simulink model "calculator"  (R2014a)
settings: Solver=VariableStepAuto  StartTime=0.0  StopTime=10.0  RelTol=1e-3
libraries: hdlsllib x43
(part 1 of 4)
settings Model: Creator=Ray  LastModifiedBy=you.r
settings DataIOCC: LimitDataPoints=off  SaveFormat=Dataset
settings OptimizationCC: LifeSpan=auto  SimCompilerOptimization=off
settings DebuggingCC: MergeDetectMultiDrivingBlocksExec=error  SolverPrmCheckMsg=none  FcnCallInpInsideContextMsg=error  FrameProcessingCompatibilityMsg=error  SFUnexpectedBacktrackingDiag=error  SFNoUnconditionalDefaultTransitionDiag=error
settings HardwareCC: ProdBitPerPointer=64  ProdLargestAtomicFloat=Float  ProdIntDivRoundTo=Zero  ProdEndianess=LittleEndian  ProdWordSize=64  ProdHWDeviceType=Intel->x86-64 (Windows64)
settings ModelReferenceCC: PropagateSignalLabelsOutOfModel=on
settings RTWCC: RTWCompilerOptimization=off
settings GRTTargetCC: TargetLangStandard=C99 (ISO)  GeneratePreprocessorConditionals=Use local settings

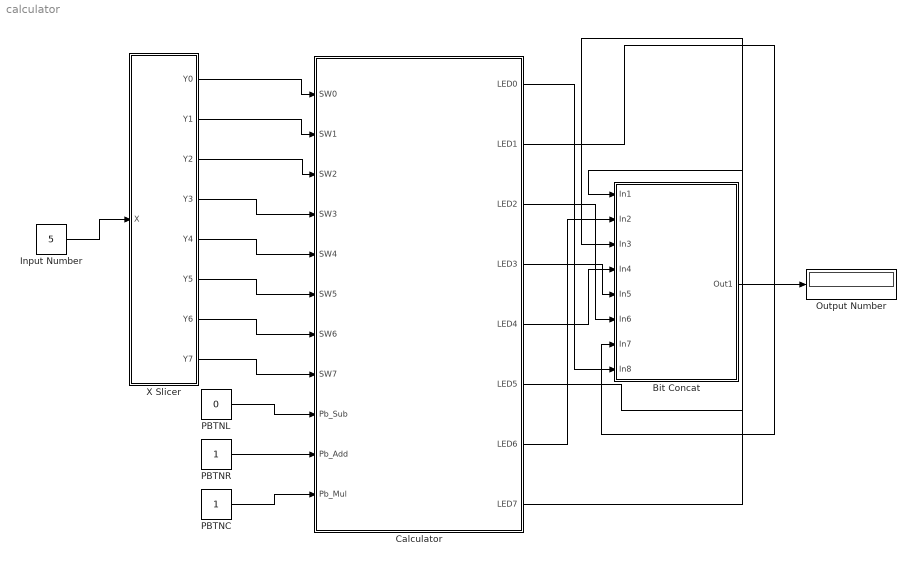
== system calculator ==
  Bit Concat : Subsystem
  Calculator : Subsystem  TreatAsAtomicUnit=on
  Input Number : Constant  Value=5  OutDataTypeStr=uint8  SampleTime=-1
  Output Number : Display
  PBTNC : Constant  OutDataTypeStr=boolean  SampleTime=1
  PBTNL : Constant  Value=0  OutDataTypeStr=boolean  SampleTime=1
  PBTNR : Constant  OutDataTypeStr=boolean  SampleTime=1
  X Slicer : Subsystem
  wires:
  Input Number/1 -> X Slicer/1(X)
  X Slicer/8(Y7) -> Calculator/8(SW7)
  X Slicer/7(Y6) -> Calculator/7(SW6)
  X Slicer/6(Y5) -> Calculator/6(SW5)
  X Slicer/5(Y4) -> Calculator/5(SW4)
  X Slicer/4(Y3) -> Calculator/4(SW3)
  X Slicer/3(Y2) -> Calculator/3(SW2)
  X Slicer/2(Y1) -> Calculator/2(SW1)
  X Slicer/1(Y0) -> Calculator/1(SW0)
  Calculator/8(LED7) -> Bit Concat/1(In1)
  Calculator/1(LED0) -> Bit Concat/8(In8)
  Calculator/2(LED1) -> Bit Concat/7(In7)
  Calculator/3(LED2) -> Bit Concat/6(In6)
  Calculator/4(LED3) -> Bit Concat/5(In5)
  Calculator/5(LED4) -> Bit Concat/4(In4)
  Calculator/6(LED5) -> Bit Concat/3(In3)
  Calculator/7(LED6) -> Bit Concat/2(In2)
  Bit Concat/1(Out1) -> Output Number/1
  PBTNR/1 -> Calculator/10(Pb_Add)
  PBTNC/1 -> Calculator/11(Pb_Mul)
  PBTNL/1 -> Calculator/9(Pb_Sub)

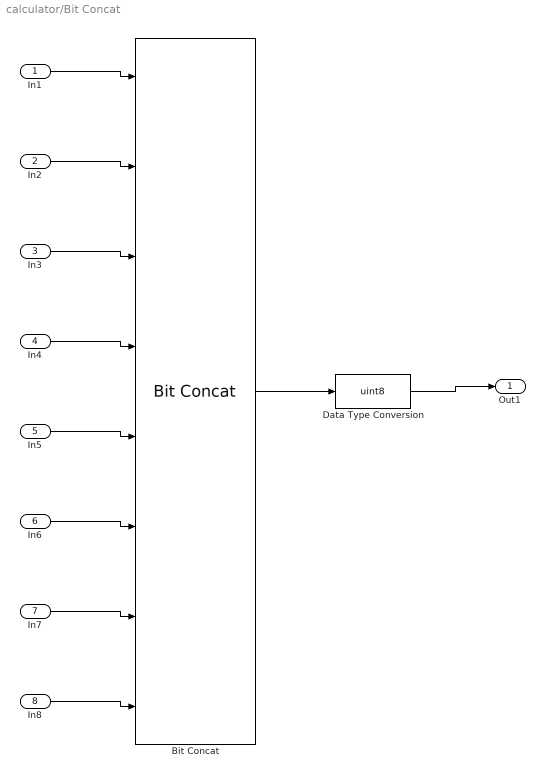
== system calculator/Bit Concat ==
  In1 : Inport
  In2 : Inport  Port=2
  In3 : Inport  Port=3
  In4 : Inport  Port=4
  In5 : Inport  Port=5
  In6 : Inport  Port=6
  In7 : Inport  Port=7
  In8 : Inport  Port=8
  Bit Concat : hdlsllib/HDL Operations/Bit Concat  numInputs=8
  Data Type Conversion : DataTypeConversion  OutDataTypeStr=uint8
  Out1 : Outport  OutDataTypeStr=uint8
  wires:
  Data Type Conversion/1 -> Out1/1
  Bit Concat/1 -> Data Type Conversion/1
  In6/1 -> Bit Concat/6
  In8/1 -> Bit Concat/8
  In1/1 -> Bit Concat/1
  In3/1 -> Bit Concat/3
  In5/1 -> Bit Concat/5
  In7/1 -> Bit Concat/7
  In4/1 -> Bit Concat/4
  In2/1 -> Bit Concat/2

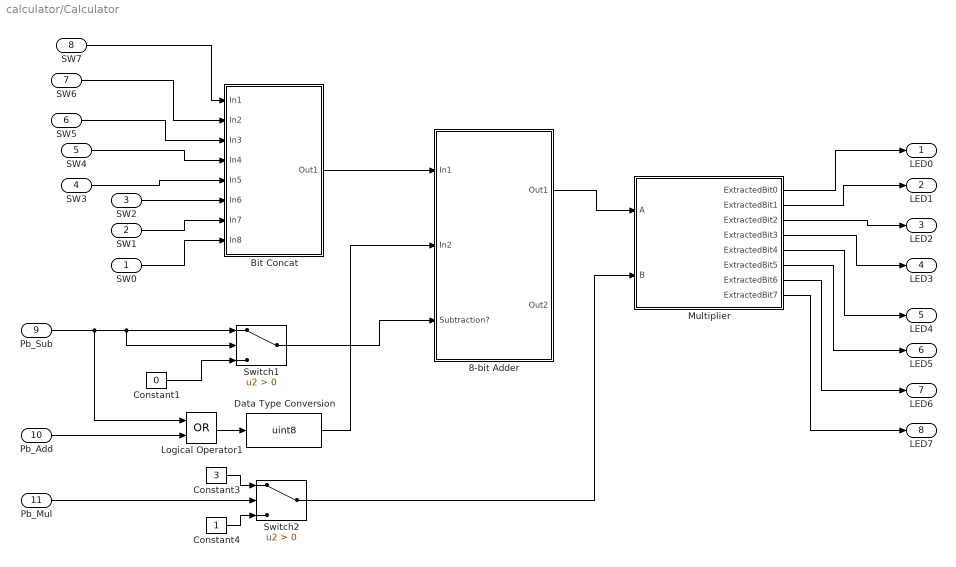
== system calculator/Calculator ==
  SW0 : Inport  OutDataTypeStr=boolean  SampleTime=1
  SW1 : Inport  Port=2  OutDataTypeStr=boolean  SampleTime=1
  SW2 : Inport  Port=3  OutDataTypeStr=boolean  SampleTime=1
  SW3 : Inport  Port=4  OutDataTypeStr=boolean  SampleTime=1
  SW4 : Inport  Port=5  OutDataTypeStr=boolean  SampleTime=1
  SW5 : Inport  Port=6  OutDataTypeStr=boolean  SampleTime=1
  SW6 : Inport  Port=7  OutDataTypeStr=boolean  SampleTime=1
  SW7 : Inport  Port=8  OutDataTypeStr=boolean  SampleTime=1
  Pb_Sub : Inport  Port=9  OutDataTypeStr=boolean  SampleTime=1
  Pb_Add : Inport  Port=10  OutDataTypeStr=boolean  SampleTime=1
  Pb_Mul : Inport  Port=11  OutDataTypeStr=boolean  SampleTime=1
  8-bit Adder : Subsystem
  Bit Concat : Subsystem
  Constant1 : Constant  Value=0  OutDataTypeStr=boolean  SampleTime=1
  Constant3 : Constant  Value=3  OutDataTypeStr=uint8  SampleTime=1
  Constant4 : Constant  OutDataTypeStr=boolean  SampleTime=1
  Data Type Conversion : DataTypeConversion  OutDataTypeStr=uint8
  Logical Operator1 : Logic  Operator=OR  AllPortsSameDT=off  OutDataTypeStr=boolean
  Multiplier : Subsystem
  Switch1 : Switch  Criteria=u2 > Threshold
  Switch2 : Switch  Criteria=u2 > Threshold  OutDataTypeStr=uint8
  LED0 : Outport  SampleTime=1
  LED1 : Outport  Port=2  SampleTime=1
  LED2 : Outport  Port=3  SampleTime=1
  LED3 : Outport  Port=4  SampleTime=1
  LED4 : Outport  Port=5  SampleTime=1
  LED5 : Outport  Port=6  SampleTime=1
  LED6 : Outport  Port=7  SampleTime=1
  LED7 : Outport  Port=8  SampleTime=1
  wires:
  Pb_Sub/1 -> Switch1/2, Switch1/1, Logical Operator1/1
  Pb_Mul/1 -> Switch2/2
  Pb_Add/1 -> Logical Operator1/2
  Bit Concat/1(Out1) -> 8-bit Adder/1(In1)
  Constant3/1 -> Switch2/1
  Switch2/1 -> Multiplier/2(B)
  Constant4/1 -> Switch2/3
  Constant1/1 -> Switch1/3
  Data Type Conversion/1 -> 8-bit Adder/2(In2)
  Logical Operator1/1 -> Data Type Conversion/1
  Multiplier/2(ExtractedBit1) -> LED1/1
  Multiplier/3(ExtractedBit2) -> LED2/1
  Multiplier/1(ExtractedBit0) -> LED0/1
  Multiplier/4(ExtractedBit3) -> LED3/1
  Multiplier/5(ExtractedBit4) -> LED4/1
  Multiplier/7(ExtractedBit6) -> LED6/1
  Multiplier/6(ExtractedBit5) -> LED5/1
  Multiplier/8(ExtractedBit7) -> LED7/1
  Switch1/1 -> 8-bit Adder/3("Subtraction? ")
  8-bit Adder/1(Out1) -> Multiplier/1(A)
  SW2/1 -> Bit Concat/6(In6)
  SW3/1 -> Bit Concat/5(In5)
  SW1/1 -> Bit Concat/7(In7)
  SW0/1 -> Bit Concat/8(In8)
  SW4/1 -> Bit Concat/4(In4)
  SW5/1 -> Bit Concat/3(In3)
  SW6/1 -> Bit Concat/2(In2)
  SW7/1 -> Bit Concat/1(In1)

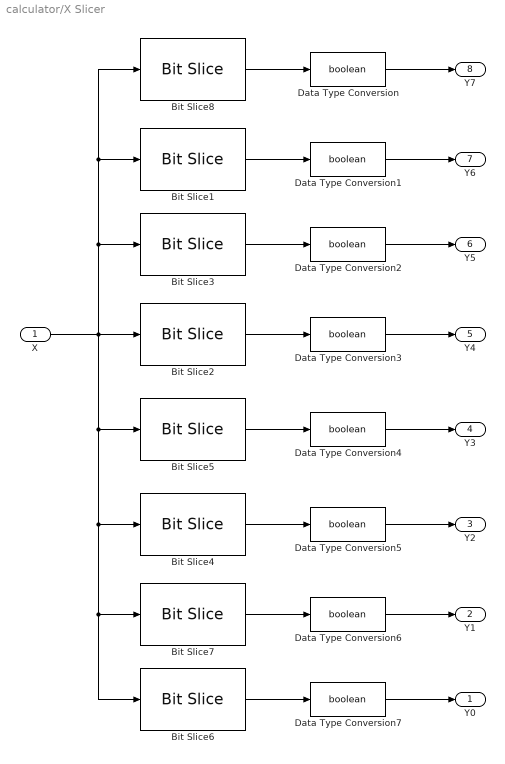
== system calculator/X Slicer ==
  X : Inport  OutDataTypeStr=uint8  SampleTime=1
  Bit Slice1 : hdlsllib/HDL Operations/Bit Slice  lidx=6  ridx=6
  Bit Slice2 : hdlsllib/HDL Operations/Bit Slice  lidx=4  ridx=4
  Bit Slice3 : hdlsllib/HDL Operations/Bit Slice  lidx=5  ridx=5
  Bit Slice4 : hdlsllib/HDL Operations/Bit Slice  lidx=2  ridx=2
  Bit Slice5 : hdlsllib/HDL Operations/Bit Slice  lidx=3  ridx=3
  Bit Slice6 : hdlsllib/HDL Operations/Bit Slice  lidx=0  ridx=0
  Bit Slice7 : hdlsllib/HDL Operations/Bit Slice  lidx=1  ridx=1
  Bit Slice8 : hdlsllib/HDL Operations/Bit Slice  lidx=7  ridx=7
  Data Type Conversion{,1..7} (8 alike) : DataTypeConversion  OutDataTypeStr=boolean
  Y0 : Outport
  Y1 : Outport  Port=2
  Y2 : Outport  Port=3
  Y3 : Outport  Port=4
  Y4 : Outport  Port=5
  Y5 : Outport  Port=6
  Y6 : Outport  Port=7
  Y7 : Outport  Port=8
  wires:
  X/1 -> Bit Slice2/1, Bit Slice5/1, Bit Slice4/1, Bit Slice7/1, Bit Slice6/1, Bit Slice3/1, Bit Slice1/1, Bit Slice8/1
  Data Type Conversion/1 -> Y7/1
  Data Type Conversion1/1 -> Y6/1
  Bit Slice3/1 -> Data Type Conversion2/1
  Bit Slice2/1 -> Data Type Conversion3/1
  Bit Slice5/1 -> Data Type Conversion4/1
  Data Type Conversion6/1 -> Y1/1
  Bit Slice8/1 -> Data Type Conversion/1
  Bit Slice1/1 -> Data Type Conversion1/1
  Bit Slice7/1 -> Data Type Conversion6/1
  Data Type Conversion7/1 -> Y0/1
  Bit Slice6/1 -> Data Type Conversion7/1
  Bit Slice4/1 -> Data Type Conversion5/1
  Data Type Conversion2/1 -> Y5/1
  Data Type Conversion3/1 -> Y4/1
  Data Type Conversion4/1 -> Y3/1
  Data Type Conversion5/1 -> Y2/1

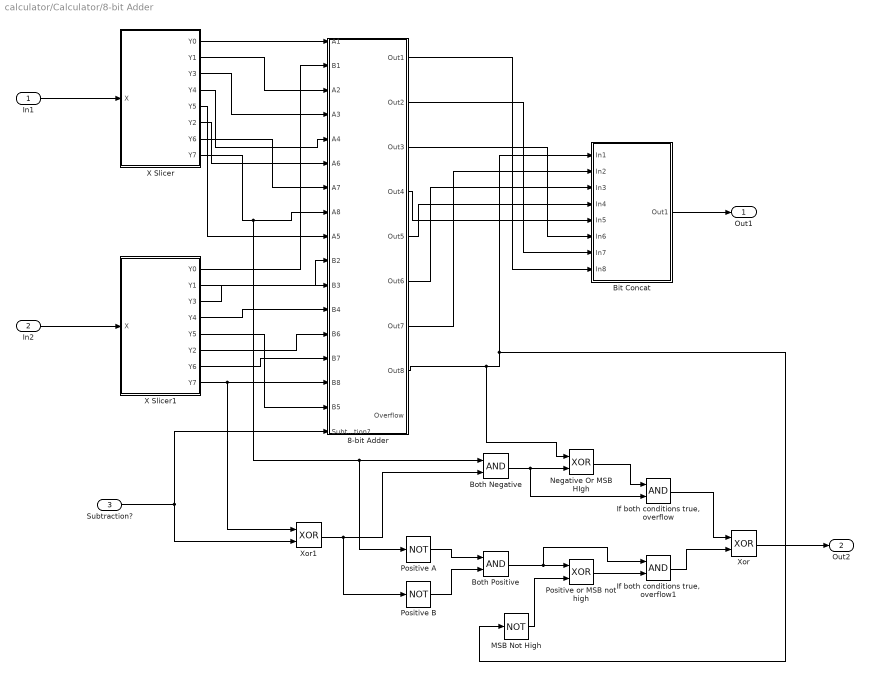
== system calculator/Calculator/8-bit Adder ==
  In1 : Inport  OutDataTypeStr=uint8
  In2 : Inport  Port=2  OutDataTypeStr=uint8
  "Subtraction? " : Inport  Port=3
  8-bit Adder : Subsystem
  Bit Concat : Subsystem
  Both Negative : Logic  AllPortsSameDT=off  OutDataTypeStr=boolean
  Both Positive : Logic  AllPortsSameDT=off  OutDataTypeStr=boolean
  "If both conditions true, overflow" : Logic  AllPortsSameDT=off  OutDataTypeStr=boolean
  "If both conditions true, overflow1" : Logic  AllPortsSameDT=off  OutDataTypeStr=boolean
  MSB Not High : Logic  Operator=NOT  AllPortsSameDT=off  OutDataTypeStr=boolean
  Negative Or MSB HIgh : Logic  Operator=XOR  AllPortsSameDT=off  OutDataTypeStr=boolean
  Positive A : Logic  Operator=NOT  AllPortsSameDT=off  OutDataTypeStr=boolean
  Positive B : Logic  Operator=NOT  AllPortsSameDT=off  OutDataTypeStr=boolean
  Positive or MSB not high : Logic  Operator=XOR  AllPortsSameDT=off  OutDataTypeStr=boolean
  X Slicer : Subsystem
  X Slicer1 : Subsystem
  Xor : Logic  Operator=XOR  AllPortsSameDT=off  OutDataTypeStr=boolean
  Xor1 : Logic  Operator=XOR  AllPortsSameDT=off  OutDataTypeStr=boolean
  Out1 : Outport
  Out2 : Outport  Port=2
  wires:
  Bit Concat/1(Out1) -> Out1/1
  In1/1 -> X Slicer/1(X)
  In2/1 -> X Slicer1/1(X)
  8-bit Adder/8(Out8) -> Negative Or MSB HIgh/1, MSB Not High/1, Bit Concat/1(In1)
  8-bit Adder/7(Out7) -> Bit Concat/2(In2)
  8-bit Adder/6(Out6) -> Bit Concat/3(In3)
  8-bit Adder/5(Out5) -> Bit Concat/4(In4)
  8-bit Adder/4(Out4) -> Bit Concat/5(In5)
  8-bit Adder/3(Out3) -> Bit Concat/6(In6)
  8-bit Adder/2(Out2) -> Bit Concat/7(In7)
  8-bit Adder/1(Out1) -> Bit Concat/8(In8)
  X Slicer/1(Y0) -> 8-bit Adder/1(A1)
  X Slicer/2(Y1) -> 8-bit Adder/3(A2)
  X Slicer/3(Y3) -> 8-bit Adder/4(A3)
  X Slicer/4(Y4) -> 8-bit Adder/5(A4)
  X Slicer/5(Y5) -> 8-bit Adder/9(A5)
  X Slicer/6(Y2) -> 8-bit Adder/6(A6)
  X Slicer/7(Y6) -> 8-bit Adder/7(A7)
  X Slicer1/1(Y0) -> 8-bit Adder/2(B1)
  X Slicer1/2(Y1) -> 8-bit Adder/10(B2)
  X Slicer1/3(Y3) -> 8-bit Adder/11(B3)
  X Slicer1/4(Y4) -> 8-bit Adder/12(B4)
  X Slicer1/5(Y5) -> 8-bit Adder/16(B5)
  X Slicer1/6(Y2) -> 8-bit Adder/13(B6)
  X Slicer1/7(Y6) -> 8-bit Adder/14(B7)
  X Slicer1/8(Y7) -> Xor1/1, 8-bit Adder/15(B8)
  Both Negative/1 -> "If both conditions true, overflow"/2, Negative Or MSB HIgh/2
  Negative Or MSB HIgh/1 -> "If both conditions true, overflow"/1
  X Slicer/8(Y7) -> Positive A/1, Both Negative/1, 8-bit Adder/8(A8)
  Positive A/1 -> Both Positive/1
  Positive B/1 -> Both Positive/2
  Both Positive/1 -> "If both conditions true, overflow1"/1, Positive or MSB not high/1
  MSB Not High/1 -> Positive or MSB not high/2
  Positive or MSB not high/1 -> "If both conditions true, overflow1"/2
  Xor/1 -> Out2/1
  "If both conditions true, overflow1"/1 -> Xor/2
  "If both conditions true, overflow"/1 -> Xor/1
  "Subtraction? "/1 -> 8-bit Adder/17(Subtraction?), Xor1/2
  Xor1/1 -> Positive B/1, Both Negative/2

== system calculator/Calculator/Bit Concat ==
  In1 : Inport
  In2 : Inport  Port=2
  In3 : Inport  Port=3
  In4 : Inport  Port=4
  In5 : Inport  Port=5
  In6 : Inport  Port=6
  In7 : Inport  Port=7
  In8 : Inport  Port=8
  Bit Concat1 : hdlsllib/HDL Operations/Bit Concat  numInputs=8
  Data Type Conversion : DataTypeConversion  OutDataTypeStr=uint8
  Out1 : Outport  OutDataTypeStr=uint8
  wires:
  Data Type Conversion/1 -> Out1/1
  Bit Concat1/1 -> Data Type Conversion/1
  In5/1 -> Bit Concat1/5
  In6/1 -> Bit Concat1/6
  In4/1 -> Bit Concat1/4
  In3/1 -> Bit Concat1/3
  In7/1 -> Bit Concat1/7
  In8/1 -> Bit Concat1/8
  In2/1 -> Bit Concat1/2
  In1/1 -> Bit Concat1/1

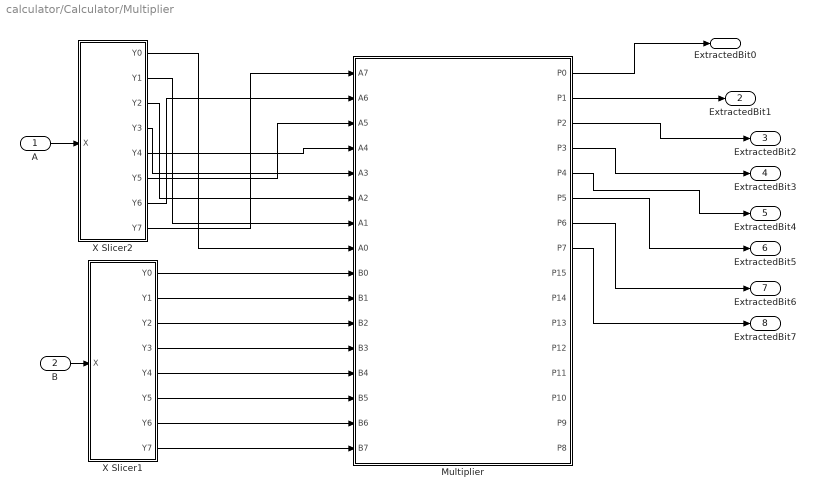
== system calculator/Calculator/Multiplier ==
  A : Inport  OutDataTypeStr=uint8
  B : Inport  Port=2  OutDataTypeStr=uint8
  Multiplier : Subsystem
  X Slicer1 : Subsystem
  X Slicer2 : Subsystem
  ExtractedBit0 : Outport  SampleTime=1
  ExtractedBit1 : Outport  Port=2  SampleTime=1
  ExtractedBit2 : Outport  Port=3  SampleTime=1
  ExtractedBit3 : Outport  Port=4  SampleTime=1
  ExtractedBit4 : Outport  Port=5  SampleTime=1
  ExtractedBit5 : Outport  Port=6  SampleTime=1
  ExtractedBit6 : Outport  Port=7  SampleTime=1
  ExtractedBit7 : Outport  Port=8  SampleTime=1
  wires:
  B/1 -> X Slicer1/1(X)
  A/1 -> X Slicer2/1(X)
  X Slicer1/1(Y0) -> Multiplier/9(B0)
  X Slicer1/2(Y1) -> Multiplier/10(B1)
  X Slicer1/3(Y2) -> Multiplier/11(B2)
  X Slicer1/4(Y3) -> Multiplier/12(B3)
  X Slicer1/5(Y4) -> Multiplier/13(B4)
  X Slicer1/6(Y5) -> Multiplier/14(B5)
  X Slicer1/7(Y6) -> Multiplier/15(B6)
  X Slicer1/8(Y7) -> Multiplier/16(B7)
  Multiplier/1(P0) -> ExtractedBit0/1
  Multiplier/2(P1) -> ExtractedBit1/1
  Multiplier/3(P2) -> ExtractedBit2/1
  Multiplier/4(P3) -> ExtractedBit3/1
  Multiplier/5(P4) -> ExtractedBit4/1
  Multiplier/6(P5) -> ExtractedBit5/1
  Multiplier/7(P6) -> ExtractedBit6/1
  Multiplier/8(P7) -> ExtractedBit7/1
  X Slicer2/8(Y7) -> Multiplier/1(A7)
  X Slicer2/1(Y0) -> Multiplier/8(A0)
  X Slicer2/2(Y1) -> Multiplier/7(A1)
  X Slicer2/3(Y2) -> Multiplier/6(A2)
  X Slicer2/4(Y3) -> Multiplier/5(A3)
  X Slicer2/5(Y4) -> Multiplier/4(A4)
  X Slicer2/6(Y5) -> Multiplier/3(A5)
  X Slicer2/7(Y6) -> Multiplier/2(A6)

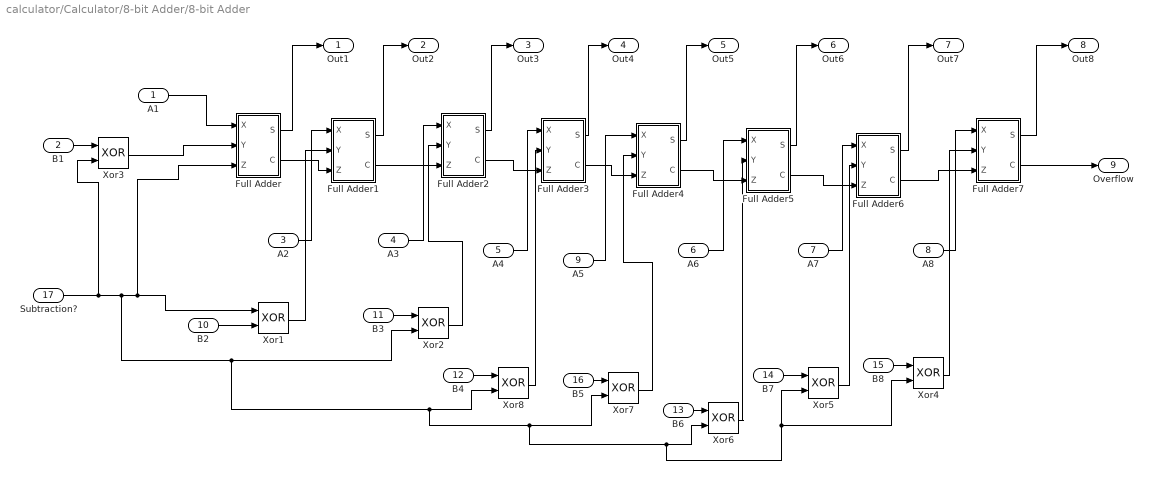
== system calculator/Calculator/8-bit Adder/8-bit Adder ==
  A1 : Inport
  B1 : Inport  Port=2
  A2 : Inport  Port=3
  A3 : Inport  Port=4
  A4 : Inport  Port=5
  A6 : Inport  Port=6
  A7 : Inport  Port=7
  A8 : Inport  Port=8
  A5 : Inport  Port=9
  B2 : Inport  Port=10
  B3 : Inport  Port=11
  B4 : Inport  Port=12
  B6 : Inport  Port=13
  B7 : Inport  Port=14
  B8 : Inport  Port=15
  B5 : Inport  Port=16
  Subtraction? : Inport  Port=17  OutDataTypeStr=boolean
  Full Adder : Subsystem
  Full Adder1 : Subsystem
  Full Adder2 : Subsystem
  Full Adder3 : Subsystem
  Full Adder4 : Subsystem
  Full Adder5 : Subsystem
  Full Adder6 : Subsystem
  Full Adder7 : Subsystem
  Xor{1..8} (8 alike) : Logic  Operator=XOR  AllPortsSameDT=off  OutDataTypeStr=boolean
  Out1 : Outport  OutDataTypeStr=boolean
  Out2 : Outport  Port=2  OutDataTypeStr=boolean
  Out3 : Outport  Port=3  OutDataTypeStr=boolean
  Out4 : Outport  Port=4  OutDataTypeStr=boolean
  Out5 : Outport  Port=5  OutDataTypeStr=boolean
  Out6 : Outport  Port=6  OutDataTypeStr=boolean
  Out7 : Outport  Port=7  OutDataTypeStr=boolean
  Out8 : Outport  Port=8  OutDataTypeStr=boolean
  Overflow : Outport  Port=9  OutDataTypeStr=boolean
  wires:
  Full Adder7/2(C) -> Overflow/1
  Full Adder5/2(C) -> Full Adder6/3(Z)
  Full Adder7/1(S) -> Out8/1
  Full Adder4/2(C) -> Full Adder5/3(Z)
  Full Adder/2(C) -> Full Adder1/3(Z)
  Full Adder6/2(C) -> Full Adder7/3(Z)
  Full Adder6/1(S) -> Out7/1
  Full Adder2/2(C) -> Full Adder3/3(Z)
  Full Adder4/1(S) -> Out5/1
  A2/1 -> Full Adder1/1(X)
  A5/1 -> Full Adder4/1(X)
  Full Adder1/1(S) -> Out2/1
  A7/1 -> Full Adder6/1(X)
  Full Adder5/1(S) -> Out6/1
  A1/1 -> Full Adder/1(X)
  A8/1 -> Full Adder7/1(X)
  A6/1 -> Full Adder5/1(X)
  A4/1 -> Full Adder3/1(X)
  Full Adder3/1(S) -> Out4/1
  Full Adder/1(S) -> Out1/1
  Full Adder1/2(C) -> Full Adder2/3(Z)
  A3/1 -> Full Adder2/1(X)
  Full Adder3/2(C) -> Full Adder4/3(Z)
  Full Adder2/1(S) -> Out3/1
  B2/1 -> Xor1/2
  Subtraction?/1 -> Xor3/2, Xor4/2, Xor5/2, Xor6/2, Xor7/2, Xor8/2, Xor2/2, Full Adder/3(Z), Xor1/1
  Xor1/1 -> Full Adder1/2(Y)
  Xor2/1 -> Full Adder2/2(Y)
  B3/1 -> Xor2/1
  B4/1 -> Xor8/1
  Xor8/1 -> Full Adder3/2(Y)
  B5/1 -> Xor7/1
  Xor7/1 -> Full Adder4/2(Y)
  B6/1 -> Xor6/1
  Xor6/1 -> Full Adder5/2(Y)
  B7/1 -> Xor5/1
  Xor5/1 -> Full Adder6/2(Y)
  Xor4/1 -> Full Adder7/2(Y)
  B8/1 -> Xor4/1
  Xor3/1 -> Full Adder/2(Y)
  B1/1 -> Xor3/1

== system calculator/Calculator/8-bit Adder/Bit Concat ==
  In1 : Inport
  In2 : Inport  Port=2
  In3 : Inport  Port=3
  In4 : Inport  Port=4
  In5 : Inport  Port=5
  In6 : Inport  Port=6
  In7 : Inport  Port=7
  In8 : Inport  Port=8
  Bit Concat : hdlsllib/HDL Operations/Bit Concat  numInputs=8
  Data Type Conversion : DataTypeConversion  OutDataTypeStr=uint8
  Out1 : Outport  OutDataTypeStr=uint8
  wires:
  Data Type Conversion/1 -> Out1/1
  Bit Concat/1 -> Data Type Conversion/1
  In6/1 -> Bit Concat/6
  In8/1 -> Bit Concat/8
  In1/1 -> Bit Concat/1
  In3/1 -> Bit Concat/3
  In5/1 -> Bit Concat/5
  In7/1 -> Bit Concat/7
  In4/1 -> Bit Concat/4
  In2/1 -> Bit Concat/2

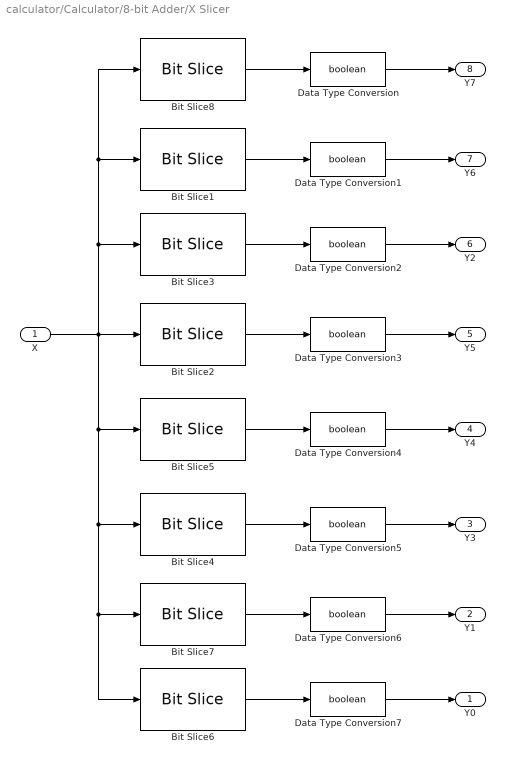
== system calculator/Calculator/8-bit Adder/X Slicer ==
  X : Inport  OutDataTypeStr=uint8  SampleTime=1
  Bit Slice1 : hdlsllib/HDL Operations/Bit Slice  lidx=6  ridx=6
  Bit Slice2 : hdlsllib/HDL Operations/Bit Slice  lidx=4  ridx=4
  Bit Slice3 : hdlsllib/HDL Operations/Bit Slice  lidx=5  ridx=5
  Bit Slice4 : hdlsllib/HDL Operations/Bit Slice  lidx=2  ridx=2
  Bit Slice5 : hdlsllib/HDL Operations/Bit Slice  lidx=3  ridx=3
  Bit Slice6 : hdlsllib/HDL Operations/Bit Slice  lidx=0  ridx=0
  Bit Slice7 : hdlsllib/HDL Operations/Bit Slice  lidx=1  ridx=1
  Bit Slice8 : hdlsllib/HDL Operations/Bit Slice  lidx=7  ridx=7
  Data Type Conversion{,1..7} (8 alike) : DataTypeConversion  OutDataTypeStr=boolean
  Y0 : Outport
  Y1 : Outport  Port=2
  Y3 : Outport  Port=3
  Y4 : Outport  Port=4
  Y5 : Outport  Port=5
  Y2 : Outport  Port=6
  Y6 : Outport  Port=7
  Y7 : Outport  Port=8
  wires:
  X/1 -> Bit Slice2/1, Bit Slice5/1, Bit Slice4/1, Bit Slice7/1, Bit Slice6/1, Bit Slice3/1, Bit Slice1/1, Bit Slice8/1
  Data Type Conversion/1 -> Y7/1
  Data Type Conversion1/1 -> Y6/1
  Bit Slice3/1 -> Data Type Conversion2/1
  Bit Slice2/1 -> Data Type Conversion3/1
  Bit Slice5/1 -> Data Type Conversion4/1
  Data Type Conversion6/1 -> Y1/1
  Bit Slice8/1 -> Data Type Conversion/1
  Bit Slice1/1 -> Data Type Conversion1/1
  Bit Slice7/1 -> Data Type Conversion6/1
  Data Type Conversion7/1 -> Y0/1
  Bit Slice6/1 -> Data Type Conversion7/1
  Bit Slice4/1 -> Data Type Conversion5/1
  Data Type Conversion2/1 -> Y2/1
  Data Type Conversion3/1 -> Y5/1
  Data Type Conversion4/1 -> Y4/1
  Data Type Conversion5/1 -> Y3/1

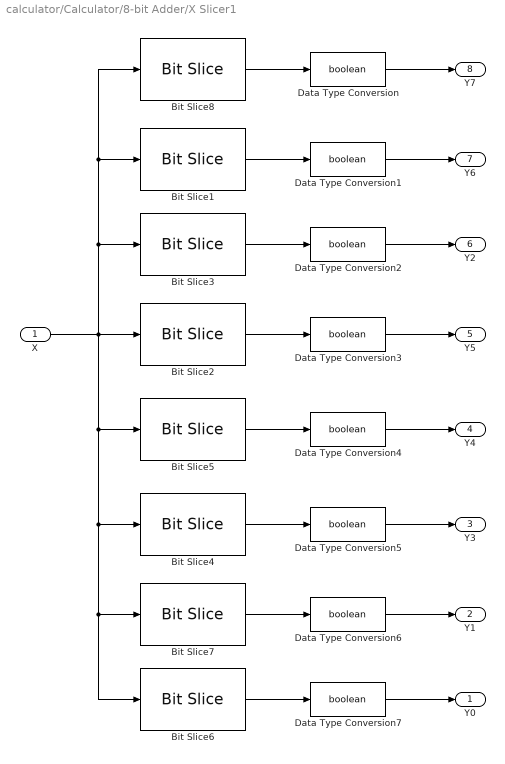
== system calculator/Calculator/8-bit Adder/X Slicer1 ==
  X : Inport  OutDataTypeStr=uint8  SampleTime=1
  Bit Slice1 : hdlsllib/HDL Operations/Bit Slice  lidx=6  ridx=6
  Bit Slice2 : hdlsllib/HDL Operations/Bit Slice  lidx=4  ridx=4
  Bit Slice3 : hdlsllib/HDL Operations/Bit Slice  lidx=5  ridx=5
  Bit Slice4 : hdlsllib/HDL Operations/Bit Slice  lidx=2  ridx=2
  Bit Slice5 : hdlsllib/HDL Operations/Bit Slice  lidx=3  ridx=3
  Bit Slice6 : hdlsllib/HDL Operations/Bit Slice  lidx=0  ridx=0
  Bit Slice7 : hdlsllib/HDL Operations/Bit Slice  lidx=1  ridx=1
  Bit Slice8 : hdlsllib/HDL Operations/Bit Slice  lidx=7  ridx=7
  Data Type Conversion{,1..7} (8 alike) : DataTypeConversion  OutDataTypeStr=boolean
  Y0 : Outport
  Y1 : Outport  Port=2
  Y3 : Outport  Port=3
  Y4 : Outport  Port=4
  Y5 : Outport  Port=5
  Y2 : Outport  Port=6
  Y6 : Outport  Port=7
  Y7 : Outport  Port=8
  wires:
  X/1 -> Bit Slice2/1, Bit Slice5/1, Bit Slice4/1, Bit Slice7/1, Bit Slice6/1, Bit Slice3/1, Bit Slice1/1, Bit Slice8/1
  Data Type Conversion/1 -> Y7/1
  Data Type Conversion1/1 -> Y6/1
  Bit Slice3/1 -> Data Type Conversion2/1
  Bit Slice2/1 -> Data Type Conversion3/1
  Bit Slice5/1 -> Data Type Conversion4/1
  Data Type Conversion6/1 -> Y1/1
  Bit Slice8/1 -> Data Type Conversion/1
  Bit Slice1/1 -> Data Type Conversion1/1
  Bit Slice7/1 -> Data Type Conversion6/1
  Data Type Conversion7/1 -> Y0/1
  Bit Slice6/1 -> Data Type Conversion7/1
  Bit Slice4/1 -> Data Type Conversion5/1
  Data Type Conversion2/1 -> Y2/1
  Data Type Conversion3/1 -> Y5/1
  Data Type Conversion4/1 -> Y4/1
  Data Type Conversion5/1 -> Y3/1

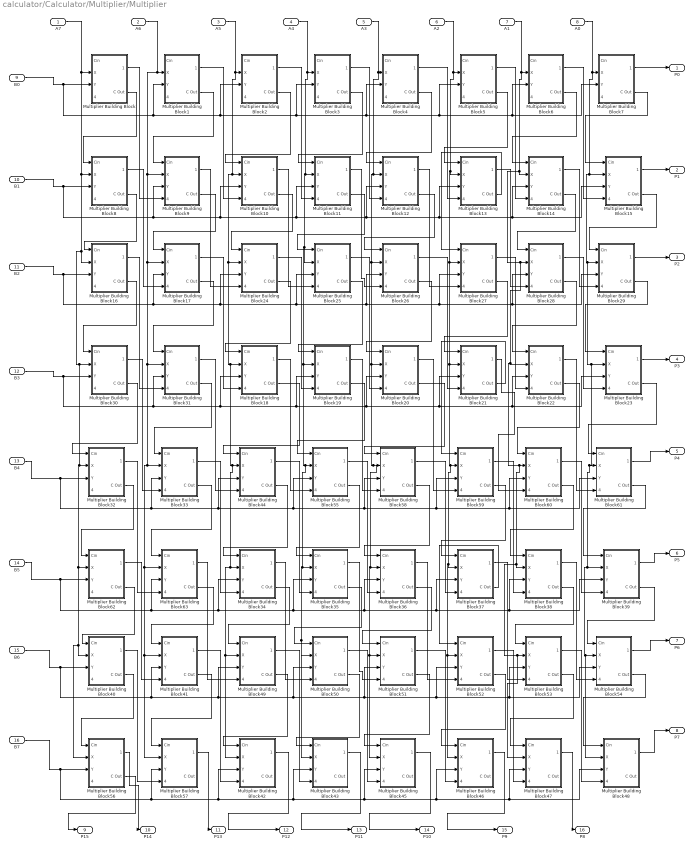
== system calculator/Calculator/Multiplier/Multiplier ==
  A7 : Inport
  A6 : Inport  Port=2
  A5 : Inport  Port=3
  A4 : Inport  Port=4
  A3 : Inport  Port=5
  A2 : Inport  Port=6
  A1 : Inport  Port=7
  A0 : Inport  Port=8
  B0 : Inport  Port=9  SampleTime=1
  B1 : Inport  Port=10  SampleTime=1
  B2 : Inport  Port=11  SampleTime=1
  B3 : Inport  Port=12  SampleTime=1
  B4 : Inport  Port=13  SampleTime=1
  B5 : Inport  Port=14  SampleTime=1
  B6 : Inport  Port=15  SampleTime=1
  B7 : Inport  Port=16  SampleTime=1
  Multiplier Building Block : Subsystem
  Multiplier Building Block1 : Subsystem
  Multiplier Building Block10 : Subsystem
  Multiplier Building Block11 : Subsystem
  Multiplier Building Block12 : Subsystem
  Multiplier Building Block13 : Subsystem
  Multiplier Building Block14 : Subsystem
  Multiplier Building Block15 : Subsystem
  Multiplier Building Block16 : Subsystem
  Multiplier Building Block17 : Subsystem
  Multiplier Building Block18 : Subsystem
  Multiplier Building Block19 : Subsystem
  Multiplier Building Block2 : Subsystem
  Multiplier Building Block20 : Subsystem
  Multiplier Building Block21 : Subsystem
  Multiplier Building Block22 : Subsystem
  Multiplier Building Block23 : Subsystem
  Multiplier Building Block24 : Subsystem
  Multiplier Building Block25 : Subsystem
  Multiplier Building Block26 : Subsystem
  Multiplier Building Block27 : Subsystem
  Multiplier Building Block28 : Subsystem
  Multiplier Building Block29 : Subsystem
  Multiplier Building Block3 : Subsystem
  Multiplier Building Block30 : Subsystem
  Multiplier Building Block31 : Subsystem
  Multiplier Building Block32 : Subsystem
  Multiplier Building Block33 : Subsystem
  Multiplier Building Block34 : Subsystem
  Multiplier Building Block35 : Subsystem
  Multiplier Building Block36 : Subsystem
  Multiplier Building Block37 : Subsystem
  Multiplier Building Block38 : Subsystem
  Multiplier Building Block39 : Subsystem
  Multiplier Building Block4 : Subsystem
  Multiplier Building Block40 : Subsystem
  Multiplier Building Block41 : Subsystem
  Multiplier Building Block42 : Subsystem
  Multiplier Building Block43 : Subsystem
  Multiplier Building Block44 : Subsystem
  Multiplier Building Block45 : Subsystem
  Multiplier Building Block46 : Subsystem
  Multiplier Building Block47 : Subsystem
  Multiplier Building Block48 : Subsystem
  Multiplier Building Block49 : Subsystem
  Multiplier Building Block5 : Subsystem
  Multiplier Building Block50 : Subsystem
  Multiplier Building Block51 : Subsystem
  Multiplier Building Block52 : Subsystem
  Multiplier Building Block53 : Subsystem
  Multiplier Building Block54 : Subsystem
  Multiplier Building Block55 : Subsystem
  Multiplier Building Block56 : Subsystem
  Multiplier Building Block57 : Subsystem
  Multiplier Building Block58 : Subsystem
  Multiplier Building Block59 : Subsystem
  Multiplier Building Block6 : Subsystem
  Multiplier Building Block60 : Subsystem
  Multiplier Building Block61 : Subsystem
  Multiplier Building Block62 : Subsystem
  Multiplier Building Block63 : Subsystem
  Multiplier Building Block7 : Subsystem
  Multiplier Building Block8 : Subsystem
  Multiplier Building Block9 : Subsystem
  P0 : Outport
  P1 : Outport  Port=2
  P2 : Outport  Port=3
  P3 : Outport  Port=4
  P4 : Outport  Port=5
  P5 : Outport  Port=6
  P6 : Outport  Port=7
  P7 : Outport  Port=8
  P15 : Outport  Port=9
  P14 : Outport  Port=10
  P13 : Outport  Port=11
  P12 : Outport  Port=12
  P11 : Outport  Port=13
  P10 : Outport  Port=14
  P9 : Outport  Port=15
  P8 : Outport  Port=16
  wires:
  Multiplier Building Block7/2(C Out) -> Multiplier Building Block15/1(Cin)
  Multiplier Building Block5/1(Sum Out) -> Multiplier Building Block14/4(Sum in)
  Multiplier Building Block6/1(Sum Out) -> Multiplier Building Block15/4(Sum in)
  Multiplier Building Block/2(C Out) -> Multiplier Building Block8/1(Cin)
  Multiplier Building Block/1(Sum Out) -> Multiplier Building Block9/4(Sum in)
  Multiplier Building Block5/2(C Out) -> Multiplier Building Block13/1(Cin)
  Multiplier Building Block2/2(C Out) -> Multiplier Building Block10/1(Cin)
  Multiplier Building Block6/2(C Out) -> Multiplier Building Block14/1(Cin)
  Multiplier Building Block4/1(Sum Out) -> Multiplier Building Block13/4(Sum in)
  Multiplier Building Block4/2(C Out) -> Multiplier Building Block12/1(Cin)
  Multiplier Building Block3/1(Sum Out) -> Multiplier Building Block12/4(Sum in)
  Multiplier Building Block3/2(C Out) -> Multiplier Building Block11/1(Cin)
  Multiplier Building Block2/1(Sum Out) -> Multiplier Building Block11/4(Sum in)
  Multiplier Building Block1/1(Sum Out) -> Multiplier Building Block10/4(Sum in)
  Multiplier Building Block1/2(C Out) -> Multiplier Building Block9/1(Cin)
  Multiplier Building Block7/1(Sum Out) -> P0/1
  B0/1 -> Multiplier Building Block3/3(Y), Multiplier Building Block7/3(Y), Multiplier Building Block6/3(Y), Multiplier Building Block5/3(Y), Multiplier Building Block4/3(Y), Multiplier Building Block2/3(Y), Multiplier Building Block1/3(Y), Multiplier Building Block/3(Y)
  Multiplier Building Block15/1(Sum Out) -> P1/1
  B1/1 -> Multiplier Building Block11/3(Y), Multiplier Building Block15/3(Y), Multiplier Building Block14/3(Y), Multiplier Building Block13/3(Y), Multiplier Building Block12/3(Y), Multiplier Building Block10/3(Y), Multiplier Building Block9/3(Y), Multiplier Building Block8/3(Y)
  Multiplier Building Block29/2(C Out) -> Multiplier Building Block23/1(Cin)
  Multiplier Building Block27/1(Sum Out) -> Multiplier Building Block22/4(Sum in)
  Multiplier Building Block28/1(Sum Out) -> Multiplier Building Block23/4(Sum in)
  Multiplier Building Block16/2(C Out) -> Multiplier Building Block30/1(Cin)
  Multiplier Building Block16/1(Sum Out) -> Multiplier Building Block31/4(Sum in)
  Multiplier Building Block27/2(C Out) -> Multiplier Building Block21/1(Cin)
  Multiplier Building Block24/2(C Out) -> Multiplier Building Block18/1(Cin)
  Multiplier Building Block28/2(C Out) -> Multiplier Building Block22/1(Cin)
  Multiplier Building Block26/1(Sum Out) -> Multiplier Building Block21/4(Sum in)
  Multiplier Building Block26/2(C Out) -> Multiplier Building Block20/1(Cin)
  Multiplier Building Block25/1(Sum Out) -> Multiplier Building Block20/4(Sum in)
  Multiplier Building Block25/2(C Out) -> Multiplier Building Block19/1(Cin)
  Multiplier Building Block24/1(Sum Out) -> Multiplier Building Block19/4(Sum in)
  Multiplier Building Block17/1(Sum Out) -> Multiplier Building Block18/4(Sum in)
  Multiplier Building Block17/2(C Out) -> Multiplier Building Block31/1(Cin)
  Multiplier Building Block29/1(Sum Out) -> P2/1
  B2/1 -> Multiplier Building Block25/3(Y), Multiplier Building Block29/3(Y), Multiplier Building Block28/3(Y), Multiplier Building Block27/3(Y), Multiplier Building Block26/3(Y), Multiplier Building Block24/3(Y), Multiplier Building Block17/3(Y), Multiplier Building Block16/3(Y)
  Multiplier Building Block23/1(Sum Out) -> P3/1
  B3/1 -> Multiplier Building Block19/3(Y), Multiplier Building Block23/3(Y), Multiplier Building Block22/3(Y), Multiplier Building Block21/3(Y), Multiplier Building Block20/3(Y), Multiplier Building Block18/3(Y), Multiplier Building Block31/3(Y), Multiplier Building Block30/3(Y)
  Multiplier Building Block15/2(C Out) -> Multiplier Building Block29/1(Cin)
  Multiplier Building Block14/1(Sum Out) -> Multiplier Building Block29/4(Sum in)
  Multiplier Building Block14/2(C Out) -> Multiplier Building Block28/1(Cin)
  Multiplier Building Block13/1(Sum Out) -> Multiplier Building Block28/4(Sum in)
  Multiplier Building Block13/2(C Out) -> Multiplier Building Block27/1(Cin)
  Multiplier Building Block12/1(Sum Out) -> Multiplier Building Block27/4(Sum in)
  Multiplier Building Block12/2(C Out) -> Multiplier Building Block26/1(Cin)
  Multiplier Building Block11/1(Sum Out) -> Multiplier Building Block26/4(Sum in)
  Multiplier Building Block11/2(C Out) -> Multiplier Building Block25/1(Cin)
  Multiplier Building Block10/1(Sum Out) -> Multiplier Building Block25/4(Sum in)
  Multiplier Building Block10/2(C Out) -> Multiplier Building Block24/1(Cin)
  Multiplier Building Block9/1(Sum Out) -> Multiplier Building Block24/4(Sum in)
  Multiplier Building Block9/2(C Out) -> Multiplier Building Block17/1(Cin)
  Multiplier Building Block8/1(Sum Out) -> Multiplier Building Block17/4(Sum in)
  Multiplier Building Block8/2(C Out) -> Multiplier Building Block16/1(Cin)
  Multiplier Building Block61/2(C Out) -> Multiplier Building Block39/1(Cin)
  Multiplier Building Block59/1(Sum Out) -> Multiplier Building Block38/4(Sum in)
  Multiplier Building Block60/1(Sum Out) -> Multiplier Building Block39/4(Sum in)
  Multiplier Building Block32/2(C Out) -> Multiplier Building Block62/1(Cin)
  Multiplier Building Block32/1(Sum Out) -> Multiplier Building Block63/4(Sum in)
  Multiplier Building Block59/2(C Out) -> Multiplier Building Block37/1(Cin)
  Multiplier Building Block44/2(C Out) -> Multiplier Building Block34/1(Cin)
  Multiplier Building Block60/2(C Out) -> Multiplier Building Block38/1(Cin)
  Multiplier Building Block58/1(Sum Out) -> Multiplier Building Block37/4(Sum in)
  Multiplier Building Block58/2(C Out) -> Multiplier Building Block36/1(Cin)
  Multiplier Building Block55/1(Sum Out) -> Multiplier Building Block36/4(Sum in)
  Multiplier Building Block55/2(C Out) -> Multiplier Building Block35/1(Cin)
  Multiplier Building Block44/1(Sum Out) -> Multiplier Building Block35/4(Sum in)
  Multiplier Building Block33/1(Sum Out) -> Multiplier Building Block34/4(Sum in)
  Multiplier Building Block33/2(C Out) -> Multiplier Building Block63/1(Cin)
  A7/1 -> Multiplier Building Block56/2(X), Multiplier Building Block40/2(X), Multiplier Building Block62/2(X), Multiplier Building Block32/2(X), Multiplier Building Block30/2(X), Multiplier Building Block16/2(X), Multiplier Building Block8/2(X), Multiplier Building Block/2(X)
  A6/1 -> Multiplier Building Block9/2(X), Multiplier Building Block31/2(X), Multiplier Building Block33/2(X), Multiplier Building Block63/2(X), Multiplier Building Block57/2(X), Multiplier Building Block41/2(X), Multiplier Building Block17/2(X), Multiplier Building Block1/2(X)
  A5/1 -> Multiplier Building Block10/2(X), Multiplier Building Block34/2(X), Multiplier Building Block42/2(X), Multiplier Building Block49/2(X), Multiplier Building Block44/2(X), Multiplier Building Block18/2(X), Multiplier Building Block24/2(X), Multiplier Building Block2/2(X)
  A4/1 -> Multiplier Building Block11/2(X), Multiplier Building Block19/2(X), Multiplier Building Block35/2(X), Multiplier Building Block43/2(X), Multiplier Building Block50/2(X), Multiplier Building Block55/2(X), Multiplier Building Block25/2(X), Multiplier Building Block3/2(X)
  A3/1 -> Multiplier Building Block12/2(X), Multiplier Building Block20/2(X), Multiplier Building Block36/2(X), Multiplier Building Block45/2(X), Multiplier Building Block51/2(X), Multiplier Building Block58/2(X), Multiplier Building Block26/2(X), Multiplier Building Block4/2(X)
  A2/1 -> Multiplier Building Block21/2(X), Multiplier Building Block46/2(X), Multiplier Building Block52/2(X), Multiplier Building Block37/2(X), Multiplier Building Block59/2(X), Multiplier Building Block27/2(X), Multiplier Building Block13/2(X), Multiplier Building Block5/2(X)
  A0/1 -> Multiplier Building Block29/2(X), Multiplier Building Block54/2(X), Multiplier Building Block48/2(X), Multiplier Building Block39/2(X), Multiplier Building Block61/2(X), Multiplier Building Block23/2(X), Multiplier Building Block15/2(X), Multiplier Building Block7/2(X)
  A1/1 -> Multiplier Building Block47/2(X), Multiplier Building Block53/2(X), Multiplier Building Block38/2(X), Multiplier Building Block60/2(X), Multiplier Building Block22/2(X), Multiplier Building Block28/2(X), Multiplier Building Block14/2(X), Multiplier Building Block6/2(X)
  Multiplier Building Block61/1(Sum Out) -> P4/1
  B4/1 -> Multiplier Building Block55/3(Y), Multiplier Building Block61/3(Y), Multiplier Building Block60/3(Y), Multiplier Building Block59/3(Y), Multiplier Building Block58/3(Y), Multiplier Building Block44/3(Y), Multiplier Building Block33/3(Y), Multiplier Building Block32/3(Y)
  Multiplier Building Block39/1(Sum Out) -> P5/1
  B5/1 -> Multiplier Building Block35/3(Y), Multiplier Building Block39/3(Y), Multiplier Building Block38/3(Y), Multiplier Building Block37/3(Y), Multiplier Building Block36/3(Y), Multiplier Building Block34/3(Y), Multiplier Building Block63/3(Y), Multiplier Building Block62/3(Y)
  Multiplier Building Block54/2(C Out) -> Multiplier Building Block48/1(Cin)
  Multiplier Building Block52/1(Sum Out) -> Multiplier Building Block47/4(Sum in)
  Multiplier Building Block53/1(Sum Out) -> Multiplier Building Block48/4(Sum in)
  Multiplier Building Block40/2(C Out) -> Multiplier Building Block56/1(Cin)
  Multiplier Building Block40/1(Sum Out) -> Multiplier Building Block57/4(Sum in)
  Multiplier Building Block52/2(C Out) -> Multiplier Building Block46/1(Cin)
  Multiplier Building Block49/2(C Out) -> Multiplier Building Block42/1(Cin)
  Multiplier Building Block53/2(C Out) -> Multiplier Building Block47/1(Cin)
  Multiplier Building Block51/1(Sum Out) -> Multiplier Building Block46/4(Sum in)
  Multiplier Building Block51/2(C Out) -> Multiplier Building Block45/1(Cin)
  Multiplier Building Block50/1(Sum Out) -> Multiplier Building Block45/4(Sum in)
  Multiplier Building Block50/2(C Out) -> Multiplier Building Block43/1(Cin)
  Multiplier Building Block49/1(Sum Out) -> Multiplier Building Block43/4(Sum in)
  Multiplier Building Block41/1(Sum Out) -> Multiplier Building Block42/4(Sum in)
  Multiplier Building Block41/2(C Out) -> Multiplier Building Block57/1(Cin)
  Multiplier Building Block54/1(Sum Out) -> P6/1
  B6/1 -> Multiplier Building Block50/3(Y), Multiplier Building Block54/3(Y), Multiplier Building Block53/3(Y), Multiplier Building Block52/3(Y), Multiplier Building Block51/3(Y), Multiplier Building Block49/3(Y), Multiplier Building Block41/3(Y), Multiplier Building Block40/3(Y)
  Multiplier Building Block48/1(Sum Out) -> P7/1
  B7/1 -> Multiplier Building Block43/3(Y), Multiplier Building Block48/3(Y), Multiplier Building Block47/3(Y), Multiplier Building Block46/3(Y), Multiplier Building Block45/3(Y), Multiplier Building Block42/3(Y), Multiplier Building Block57/3(Y), Multiplier Building Block56/3(Y)
  Multiplier Building Block39/2(C Out) -> Multiplier Building Block54/1(Cin)
  Multiplier Building Block38/1(Sum Out) -> Multiplier Building Block54/4(Sum in)
  Multiplier Building Block38/2(C Out) -> Multiplier Building Block53/1(Cin)
  Multiplier Building Block37/1(Sum Out) -> Multiplier Building Block53/4(Sum in)
  Multiplier Building Block37/2(C Out) -> Multiplier Building Block52/1(Cin)
  Multiplier Building Block36/1(Sum Out) -> Multiplier Building Block52/4(Sum in)
  Multiplier Building Block36/2(C Out) -> Multiplier Building Block51/1(Cin)
  Multiplier Building Block35/1(Sum Out) -> Multiplier Building Block51/4(Sum in)
  Multiplier Building Block35/2(C Out) -> Multiplier Building Block50/1(Cin)
  Multiplier Building Block34/1(Sum Out) -> Multiplier Building Block50/4(Sum in)
  Multiplier Building Block34/2(C Out) -> Multiplier Building Block49/1(Cin)
  Multiplier Building Block63/1(Sum Out) -> Multiplier Building Block49/4(Sum in)
  Multiplier Building Block63/2(C Out) -> Multiplier Building Block41/1(Cin)
  Multiplier Building Block62/1(Sum Out) -> Multiplier Building Block41/4(Sum in)
  Multiplier Building Block62/2(C Out) -> Multiplier Building Block40/1(Cin)
  Multiplier Building Block23/2(C Out) -> Multiplier Building Block61/1(Cin)
  Multiplier Building Block22/1(Sum Out) -> Multiplier Building Block61/4(Sum in)
  Multiplier Building Block22/2(C Out) -> Multiplier Building Block60/1(Cin)
  Multiplier Building Block21/1(Sum Out) -> Multiplier Building Block60/4(Sum in)
  Multiplier Building Block21/2(C Out) -> Multiplier Building Block59/1(Cin)
  Multiplier Building Block20/1(Sum Out) -> Multiplier Building Block59/4(Sum in)
  Multiplier Building Block20/2(C Out) -> Multiplier Building Block58/1(Cin)
  Multiplier Building Block19/1(Sum Out) -> Multiplier Building Block58/4(Sum in)
  Multiplier Building Block19/2(C Out) -> Multiplier Building Block55/1(Cin)
  Multiplier Building Block18/1(Sum Out) -> Multiplier Building Block55/4(Sum in)
  Multiplier Building Block18/2(C Out) -> Multiplier Building Block44/1(Cin)
  Multiplier Building Block31/1(Sum Out) -> Multiplier Building Block44/4(Sum in)
  Multiplier Building Block31/2(C Out) -> Multiplier Building Block33/1(Cin)
  Multiplier Building Block30/1(Sum Out) -> Multiplier Building Block33/4(Sum in)
  Multiplier Building Block30/2(C Out) -> Multiplier Building Block32/1(Cin)
  Multiplier Building Block56/2(C Out) -> P15/1
  Multiplier Building Block56/1(Sum Out) -> P14/1
  Multiplier Building Block57/1(Sum Out) -> P13/1
  Multiplier Building Block42/1(Sum Out) -> P12/1
  Multiplier Building Block43/1(Sum Out) -> P11/1
  Multiplier Building Block45/1(Sum Out) -> P10/1
  Multiplier Building Block46/1(Sum Out) -> P9/1
  Multiplier Building Block47/1(Sum Out) -> P8/1

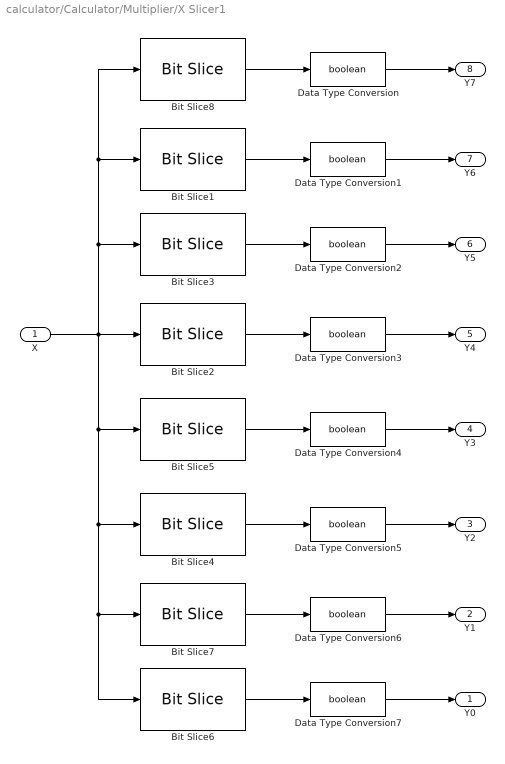
== system calculator/Calculator/Multiplier/X Slicer1 ==
  X : Inport  OutDataTypeStr=uint8  SampleTime=1
  Bit Slice1 : hdlsllib/HDL Operations/Bit Slice  lidx=6  ridx=6
  Bit Slice2 : hdlsllib/HDL Operations/Bit Slice  lidx=4  ridx=4
  Bit Slice3 : hdlsllib/HDL Operations/Bit Slice  lidx=5  ridx=5
  Bit Slice4 : hdlsllib/HDL Operations/Bit Slice  lidx=2  ridx=2
  Bit Slice5 : hdlsllib/HDL Operations/Bit Slice  lidx=3  ridx=3
  Bit Slice6 : hdlsllib/HDL Operations/Bit Slice  lidx=0  ridx=0
  Bit Slice7 : hdlsllib/HDL Operations/Bit Slice  lidx=1  ridx=1
  Bit Slice8 : hdlsllib/HDL Operations/Bit Slice  lidx=7  ridx=7
  Data Type Conversion{,1..7} (8 alike) : DataTypeConversion  OutDataTypeStr=boolean
  Y0 : Outport
  Y1 : Outport  Port=2
  Y2 : Outport  Port=3
  Y3 : Outport  Port=4
  Y4 : Outport  Port=5
  Y5 : Outport  Port=6
  Y6 : Outport  Port=7
  Y7 : Outport  Port=8
  wires:
  X/1 -> Bit Slice2/1, Bit Slice5/1, Bit Slice4/1, Bit Slice7/1, Bit Slice6/1, Bit Slice3/1, Bit Slice1/1, Bit Slice8/1
  Data Type Conversion/1 -> Y7/1
  Data Type Conversion1/1 -> Y6/1
  Bit Slice3/1 -> Data Type Conversion2/1
  Bit Slice2/1 -> Data Type Conversion3/1
  Bit Slice5/1 -> Data Type Conversion4/1
  Data Type Conversion6/1 -> Y1/1
  Bit Slice8/1 -> Data Type Conversion/1
  Bit Slice1/1 -> Data Type Conversion1/1
  Bit Slice7/1 -> Data Type Conversion6/1
  Data Type Conversion7/1 -> Y0/1
  Bit Slice6/1 -> Data Type Conversion7/1
  Bit Slice4/1 -> Data Type Conversion5/1
  Data Type Conversion2/1 -> Y5/1
  Data Type Conversion3/1 -> Y4/1
  Data Type Conversion4/1 -> Y3/1
  Data Type Conversion5/1 -> Y2/1

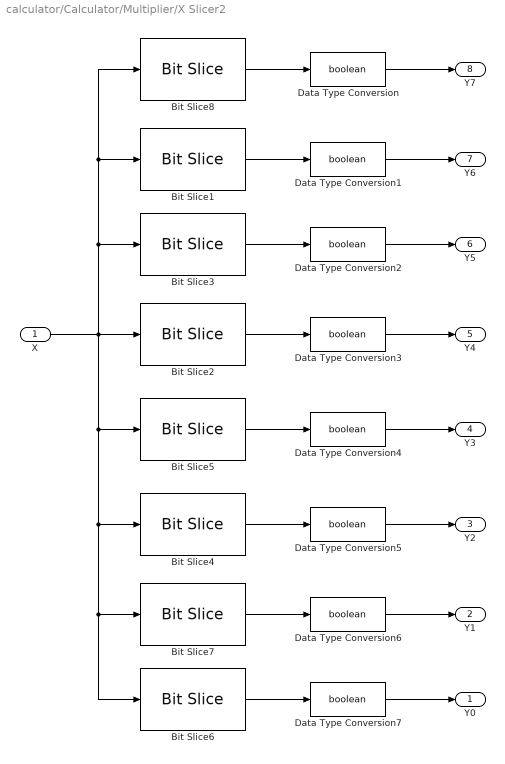
== system calculator/Calculator/Multiplier/X Slicer2 ==
  X : Inport  OutDataTypeStr=uint8  SampleTime=1
  Bit Slice1 : hdlsllib/HDL Operations/Bit Slice  lidx=6  ridx=6
  Bit Slice2 : hdlsllib/HDL Operations/Bit Slice  lidx=4  ridx=4
  Bit Slice3 : hdlsllib/HDL Operations/Bit Slice  lidx=5  ridx=5
  Bit Slice4 : hdlsllib/HDL Operations/Bit Slice  lidx=2  ridx=2
  Bit Slice5 : hdlsllib/HDL Operations/Bit Slice  lidx=3  ridx=3
  Bit Slice6 : hdlsllib/HDL Operations/Bit Slice  lidx=0  ridx=0
  Bit Slice7 : hdlsllib/HDL Operations/Bit Slice  lidx=1  ridx=1
  Bit Slice8 : hdlsllib/HDL Operations/Bit Slice  lidx=7  ridx=7
  Data Type Conversion{,1..7} (8 alike) : DataTypeConversion  OutDataTypeStr=boolean
  Y0 : Outport
  Y1 : Outport  Port=2
  Y2 : Outport  Port=3
  Y3 : Outport  Port=4
  Y4 : Outport  Port=5
  Y5 : Outport  Port=6
  Y6 : Outport  Port=7
  Y7 : Outport  Port=8
  wires:
  X/1 -> Bit Slice2/1, Bit Slice5/1, Bit Slice4/1, Bit Slice7/1, Bit Slice6/1, Bit Slice3/1, Bit Slice1/1, Bit Slice8/1
  Data Type Conversion/1 -> Y7/1
  Data Type Conversion1/1 -> Y6/1
  Bit Slice3/1 -> Data Type Conversion2/1
  Bit Slice2/1 -> Data Type Conversion3/1
  Bit Slice5/1 -> Data Type Conversion4/1
  Data Type Conversion6/1 -> Y1/1
  Bit Slice8/1 -> Data Type Conversion/1
  Bit Slice1/1 -> Data Type Conversion1/1
  Bit Slice7/1 -> Data Type Conversion6/1
  Data Type Conversion7/1 -> Y0/1
  Bit Slice6/1 -> Data Type Conversion7/1
  Bit Slice4/1 -> Data Type Conversion5/1
  Data Type Conversion2/1 -> Y5/1
  Data Type Conversion3/1 -> Y4/1
  Data Type Conversion4/1 -> Y3/1
  Data Type Conversion5/1 -> Y2/1

== system calculator/Calculator/8-bit Adder/8-bit Adder/Full Adder ==
  X : Inport
  Y : Inport  Port=2
  Z : Inport  Port=3
  Half Adder : Subsystem
  Half Adder1 : Subsystem
  OR : Logic  Operator=OR  IconShape=distinctive  AllPortsSameDT=off  OutDataTypeStr=boolean
  S : Outport
  C : Outport  Port=2
  wires:
  Half Adder1/1(Sum) -> S/1
  Half Adder/1(Sum) -> Half Adder1/1(A)
  Half Adder/2(Carry) -> OR/2
  X/1 -> Half Adder/1(A)
  Z/1 -> Half Adder1/2(B)
  OR/1 -> C/1
  Y/1 -> Half Adder/2(B)
  Half Adder1/2(Carry) -> OR/1

== system calculator/Calculator/8-bit Adder/8-bit Adder/Full Adder1 ==
  X : Inport
  Y : Inport  Port=2
  Z : Inport  Port=3
  Half Adder : Subsystem
  Half Adder1 : Subsystem
  OR : Logic  Operator=OR  IconShape=distinctive  AllPortsSameDT=off  OutDataTypeStr=boolean
  S : Outport
  C : Outport  Port=2
  wires:
  Half Adder1/1(Sum) -> S/1
  Half Adder/1(Sum) -> Half Adder1/1(A)
  Half Adder/2(Carry) -> OR/2
  X/1 -> Half Adder/1(A)
  Z/1 -> Half Adder1/2(B)
  OR/1 -> C/1
  Y/1 -> Half Adder/2(B)
  Half Adder1/2(Carry) -> OR/1

== system calculator/Calculator/8-bit Adder/8-bit Adder/Full Adder2 ==
  X : Inport
  Y : Inport  Port=2
  Z : Inport  Port=3
  Half Adder : Subsystem
  Half Adder1 : Subsystem
  OR : Logic  Operator=OR  IconShape=distinctive  AllPortsSameDT=off  OutDataTypeStr=boolean
  S : Outport
  C : Outport  Port=2
  wires:
  Half Adder1/1(Sum) -> S/1
  Half Adder/1(Sum) -> Half Adder1/1(A)
  Half Adder/2(Carry) -> OR/2
  X/1 -> Half Adder/1(A)
  Z/1 -> Half Adder1/2(B)
  OR/1 -> C/1
  Y/1 -> Half Adder/2(B)
  Half Adder1/2(Carry) -> OR/1

== system calculator/Calculator/8-bit Adder/8-bit Adder/Full Adder3 ==
  X : Inport
  Y : Inport  Port=2
  Z : Inport  Port=3
  Half Adder : Subsystem
  Half Adder1 : Subsystem
  OR : Logic  Operator=OR  IconShape=distinctive  AllPortsSameDT=off  OutDataTypeStr=boolean
  S : Outport
  C : Outport  Port=2
  wires:
  Half Adder1/1(Sum) -> S/1
  Half Adder/1(Sum) -> Half Adder1/1(A)
  Half Adder/2(Carry) -> OR/2
  X/1 -> Half Adder/1(A)
  Z/1 -> Half Adder1/2(B)
  OR/1 -> C/1
  Y/1 -> Half Adder/2(B)
  Half Adder1/2(Carry) -> OR/1

== system calculator/Calculator/8-bit Adder/8-bit Adder/Full Adder4 ==
  X : Inport
  Y : Inport  Port=2
  Z : Inport  Port=3
  Half Adder : Subsystem
  Half Adder1 : Subsystem
  OR : Logic  Operator=OR  IconShape=distinctive  AllPortsSameDT=off  OutDataTypeStr=boolean
  S : Outport
  C : Outport  Port=2
  wires:
  Half Adder1/1(Sum) -> S/1
  Half Adder/1(Sum) -> Half Adder1/1(A)
  Half Adder/2(Carry) -> OR/2
  X/1 -> Half Adder/1(A)
  Z/1 -> Half Adder1/2(B)
  OR/1 -> C/1
  Y/1 -> Half Adder/2(B)
  Half Adder1/2(Carry) -> OR/1

== system calculator/Calculator/8-bit Adder/8-bit Adder/Full Adder5 ==
  X : Inport
  Y : Inport  Port=2
  Z : Inport  Port=3
  Half Adder : Subsystem
  Half Adder1 : Subsystem
  OR : Logic  Operator=OR  IconShape=distinctive  AllPortsSameDT=off  OutDataTypeStr=boolean
  S : Outport
  C : Outport  Port=2
  wires:
  Half Adder1/1(Sum) -> S/1
  Half Adder/1(Sum) -> Half Adder1/1(A)
  Half Adder/2(Carry) -> OR/2
  X/1 -> Half Adder/1(A)
  Z/1 -> Half Adder1/2(B)
  OR/1 -> C/1
  Y/1 -> Half Adder/2(B)
  Half Adder1/2(Carry) -> OR/1

== system calculator/Calculator/8-bit Adder/8-bit Adder/Full Adder6 ==
  X : Inport
  Y : Inport  Port=2
  Z : Inport  Port=3
  Half Adder : Subsystem
  Half Adder1 : Subsystem
  OR : Logic  Operator=OR  IconShape=distinctive  AllPortsSameDT=off  OutDataTypeStr=boolean
  S : Outport
  C : Outport  Port=2
  wires:
  Half Adder1/1(Sum) -> S/1
  Half Adder/1(Sum) -> Half Adder1/1(A)
  Half Adder/2(Carry) -> OR/2
  X/1 -> Half Adder/1(A)
  Z/1 -> Half Adder1/2(B)
  OR/1 -> C/1
  Y/1 -> Half Adder/2(B)
  Half Adder1/2(Carry) -> OR/1

== system calculator/Calculator/8-bit Adder/8-bit Adder/Full Adder7 ==
  X : Inport
  Y : Inport  Port=2
  Z : Inport  Port=3
  Half Adder : Subsystem
  Half Adder1 : Subsystem
  OR : Logic  Operator=OR  IconShape=distinctive  AllPortsSameDT=off  OutDataTypeStr=boolean
  S : Outport
  C : Outport  Port=2
  wires:
  Half Adder1/1(Sum) -> S/1
  Half Adder/1(Sum) -> Half Adder1/1(A)
  Half Adder/2(Carry) -> OR/2
  X/1 -> Half Adder/1(A)
  Z/1 -> Half Adder1/2(B)
  OR/1 -> C/1
  Y/1 -> Half Adder/2(B)
  Half Adder1/2(Carry) -> OR/1

== system calculator/Calculator/Multiplier/Multiplier/Multiplier Building Block ==
  Cin : Inport
  X : Inport  Port=2
  Y : Inport  Port=3
  Sum in : Inport  Port=4
  AND : Logic  IconShape=distinctive  AllPortsSameDT=off  OutDataTypeStr=boolean
  Full Adder : Subsystem
  Sum Out : Outport
  C Out : Outport  Port=2
  wires:
  Cin/1 -> Full Adder/3(Z)
  Sum in/1 -> Full Adder/1(X)
  AND/1 -> Full Adder/2(Y)
  Full Adder/1(S) -> Sum Out/1
  Y/1 -> AND/2
  X/1 -> AND/1
  Full Adder/2(C) -> C Out/1

== system calculator/Calculator/Multiplier/Multiplier/Multiplier Building Block1 ==
  Cin : Inport
  X : Inport  Port=2
  Y : Inport  Port=3
  Sum in : Inport  Port=4
  AND : Logic  IconShape=distinctive  AllPortsSameDT=off  OutDataTypeStr=boolean
  Full Adder : Subsystem
  Sum Out : Outport
  C Out : Outport  Port=2
  wires:
  Cin/1 -> Full Adder/3(Z)
  Sum in/1 -> Full Adder/1(X)
  AND/1 -> Full Adder/2(Y)
  Full Adder/1(S) -> Sum Out/1
  Y/1 -> AND/2
  X/1 -> AND/1
  Full Adder/2(C) -> C Out/1

== system calculator/Calculator/Multiplier/Multiplier/Multiplier Building Block10 ==
  Cin : Inport
  X : Inport  Port=2
  Y : Inport  Port=3
  Sum in : Inport  Port=4
  AND : Logic  IconShape=distinctive  AllPortsSameDT=off  OutDataTypeStr=boolean
  Full Adder : Subsystem
  Sum Out : Outport
  C Out : Outport  Port=2
  wires:
  Cin/1 -> Full Adder/3(Z)
  Sum in/1 -> Full Adder/1(X)
  AND/1 -> Full Adder/2(Y)
  Full Adder/1(S) -> Sum Out/1
  Y/1 -> AND/2
  X/1 -> AND/1
  Full Adder/2(C) -> C Out/1

== system calculator/Calculator/Multiplier/Multiplier/Multiplier Building Block11 ==
  Cin : Inport
  X : Inport  Port=2
  Y : Inport  Port=3
  Sum in : Inport  Port=4
  AND : Logic  IconShape=distinctive  AllPortsSameDT=off  OutDataTypeStr=boolean
  Full Adder : Subsystem
  Sum Out : Outport
  C Out : Outport  Port=2
  wires:
  Cin/1 -> Full Adder/3(Z)
  Sum in/1 -> Full Adder/1(X)
  AND/1 -> Full Adder/2(Y)
  Full Adder/1(S) -> Sum Out/1
  Y/1 -> AND/2
  X/1 -> AND/1
  Full Adder/2(C) -> C Out/1

== system calculator/Calculator/Multiplier/Multiplier/Multiplier Building Block12 ==
  Cin : Inport
  X : Inport  Port=2
  Y : Inport  Port=3
  Sum in : Inport  Port=4
  AND : Logic  IconShape=distinctive  AllPortsSameDT=off  OutDataTypeStr=boolean
  Full Adder : Subsystem
  Sum Out : Outport
  C Out : Outport  Port=2
  wires:
  Cin/1 -> Full Adder/3(Z)
  Sum in/1 -> Full Adder/1(X)
  AND/1 -> Full Adder/2(Y)
  Full Adder/1(S) -> Sum Out/1
  Y/1 -> AND/2
  X/1 -> AND/1
  Full Adder/2(C) -> C Out/1

== system calculator/Calculator/Multiplier/Multiplier/Multiplier Building Block13 ==
  Cin : Inport
  X : Inport  Port=2
  Y : Inport  Port=3
  Sum in : Inport  Port=4
  AND : Logic  IconShape=distinctive  AllPortsSameDT=off  OutDataTypeStr=boolean
  Full Adder : Subsystem
  Sum Out : Outport
  C Out : Outport  Port=2
  wires:
  Cin/1 -> Full Adder/3(Z)
  Sum in/1 -> Full Adder/1(X)
  AND/1 -> Full Adder/2(Y)
  Full Adder/1(S) -> Sum Out/1
  Y/1 -> AND/2
  X/1 -> AND/1
  Full Adder/2(C) -> C Out/1

== system calculator/Calculator/Multiplier/Multiplier/Multiplier Building Block14 ==
  Cin : Inport
  X : Inport  Port=2
  Y : Inport  Port=3
  Sum in : Inport  Port=4
  AND : Logic  IconShape=distinctive  AllPortsSameDT=off  OutDataTypeStr=boolean
  Full Adder : Subsystem
  Sum Out : Outport
  C Out : Outport  Port=2
  wires:
  Cin/1 -> Full Adder/3(Z)
  Sum in/1 -> Full Adder/1(X)
  AND/1 -> Full Adder/2(Y)
  Full Adder/1(S) -> Sum Out/1
  Y/1 -> AND/2
  X/1 -> AND/1
  Full Adder/2(C) -> C Out/1

== system calculator/Calculator/Multiplier/Multiplier/Multiplier Building Block15 ==
  Cin : Inport
  X : Inport  Port=2
  Y : Inport  Port=3
  Sum in : Inport  Port=4
  AND : Logic  IconShape=distinctive  AllPortsSameDT=off  OutDataTypeStr=boolean
  Full Adder : Subsystem
  Sum Out : Outport
  C Out : Outport  Port=2
  wires:
  Cin/1 -> Full Adder/3(Z)
  Sum in/1 -> Full Adder/1(X)
  AND/1 -> Full Adder/2(Y)
  Full Adder/1(S) -> Sum Out/1
  Y/1 -> AND/2
  X/1 -> AND/1
  Full Adder/2(C) -> C Out/1

== system calculator/Calculator/Multiplier/Multiplier/Multiplier Building Block16 ==
  Cin : Inport
  X : Inport  Port=2
  Y : Inport  Port=3
  Sum in : Inport  Port=4
  AND : Logic  IconShape=distinctive  AllPortsSameDT=off  OutDataTypeStr=boolean
  Full Adder : Subsystem
  Sum Out : Outport
  C Out : Outport  Port=2
  wires:
  Cin/1 -> Full Adder/3(Z)
  Sum in/1 -> Full Adder/1(X)
  AND/1 -> Full Adder/2(Y)
  Full Adder/1(S) -> Sum Out/1
  Y/1 -> AND/2
  X/1 -> AND/1
  Full Adder/2(C) -> C Out/1

== system calculator/Calculator/Multiplier/Multiplier/Multiplier Building Block17 ==
  Cin : Inport
  X : Inport  Port=2
  Y : Inport  Port=3
  Sum in : Inport  Port=4
  AND : Logic  IconShape=distinctive  AllPortsSameDT=off  OutDataTypeStr=boolean
  Full Adder : Subsystem
  Sum Out : Outport
  C Out : Outport  Port=2
  wires:
  Cin/1 -> Full Adder/3(Z)
  Sum in/1 -> Full Adder/1(X)
  AND/1 -> Full Adder/2(Y)
  Full Adder/1(S) -> Sum Out/1
  Y/1 -> AND/2
  X/1 -> AND/1
  Full Adder/2(C) -> C Out/1

== system calculator/Calculator/Multiplier/Multiplier/Multiplier Building Block18 ==
  Cin : Inport
  X : Inport  Port=2
  Y : Inport  Port=3
  Sum in : Inport  Port=4
  AND : Logic  IconShape=distinctive  AllPortsSameDT=off  OutDataTypeStr=boolean
  Full Adder : Subsystem
  Sum Out : Outport
  C Out : Outport  Port=2
  wires:
  Cin/1 -> Full Adder/3(Z)
  Sum in/1 -> Full Adder/1(X)
  AND/1 -> Full Adder/2(Y)
  Full Adder/1(S) -> Sum Out/1
  Y/1 -> AND/2
  X/1 -> AND/1
  Full Adder/2(C) -> C Out/1

== system calculator/Calculator/Multiplier/Multiplier/Multiplier Building Block19 ==
  Cin : Inport
  X : Inport  Port=2
  Y : Inport  Port=3
  Sum in : Inport  Port=4
  AND : Logic  IconShape=distinctive  AllPortsSameDT=off  OutDataTypeStr=boolean
  Full Adder : Subsystem
  Sum Out : Outport
  C Out : Outport  Port=2
  wires:
  Cin/1 -> Full Adder/3(Z)
  Sum in/1 -> Full Adder/1(X)
  AND/1 -> Full Adder/2(Y)
  Full Adder/1(S) -> Sum Out/1
  Y/1 -> AND/2
  X/1 -> AND/1
  Full Adder/2(C) -> C Out/1

== system calculator/Calculator/Multiplier/Multiplier/Multiplier Building Block2 ==
  Cin : Inport
  X : Inport  Port=2
  Y : Inport  Port=3
  Sum in : Inport  Port=4
  AND : Logic  IconShape=distinctive  AllPortsSameDT=off  OutDataTypeStr=boolean
  Full Adder : Subsystem
  Sum Out : Outport
  C Out : Outport  Port=2
  wires:
  Cin/1 -> Full Adder/3(Z)
  Sum in/1 -> Full Adder/1(X)
  AND/1 -> Full Adder/2(Y)
  Full Adder/1(S) -> Sum Out/1
  Y/1 -> AND/2
  X/1 -> AND/1
  Full Adder/2(C) -> C Out/1
